simulink model "verify_Storage_Type_11_mdl_electric"  (R2018b)
settings: Solver=VariableStepAuto  StartTime=0  StopTime=9000  MaxStep=60  RelTol=1e-3  EnableMultiTasking=on
undefined symbols (not defined in the file or in its folder): path_carnot
libraries: carnot x10, simulink x5
settings Model: DEBUGGLOBALLEVEL=DEBUGLEVEL  DEBUGMAXTOTALWARNINGS=0  DEBUGMAXCONSECUTIVEWARNINGS=0  DEBUGWRITETOFILE=0  DEBUGFILENAME='error.txt'  Creator=drhf  LastModifiedBy=P41573
settings DataIOCC: SaveFormat=Array
settings OptimizationCC: ExpressionDepthLimit=2147483647  LifeSpan=inf
settings DebuggingCC: UnderspecifiedInitializationDetection=Classic  MergeDetectMultiDrivingBlocksExec=none  SolverPrmCheckMsg=warning  FcnCallInpInsideContextMsg=warning  StateNameClashWarn=warning  SFUnexpectedBacktrackingDiag=warning  SFNoUnconditionalDefaultTransitionDiag=warning  SFExecutionAtInitializationDiag=none
settings HardwareCC: ProdBitPerPointer=32  ProdBitPerSizeT=32  ProdBitPerPtrDiffT=32  ProdLargestAtomicFloat=None  ProdIntDivRoundTo=Undefined  ProdEndianess=Unspecified  ProdWordSize=32  ProdHWDeviceType=32-bit Generic
settings ModelReferenceCC: PropagateSignalLabelsOutOfModel=off
settings SFSimCC: SimUseLocalCustomCode=off
settings RTWCC: RTWUseLocalCustomCode=off
settings CodeAppCC: StateflowObjectComments=on
settings GRTTargetCC: TargetLangStandard=C89/C90 (ANSI)  GeneratePreprocessorConditionals=Disable all  CombineOutputUpdateFcns=off  GRTInterface=on
settings ConfigComp: CovMetricSettings=dw  CovHtmlReporting=on  CovSaveCumulativeToWorkspaceVar=on  CovSaveSingleToWorkspaceVar=on  CovExternalEMLEnable=off

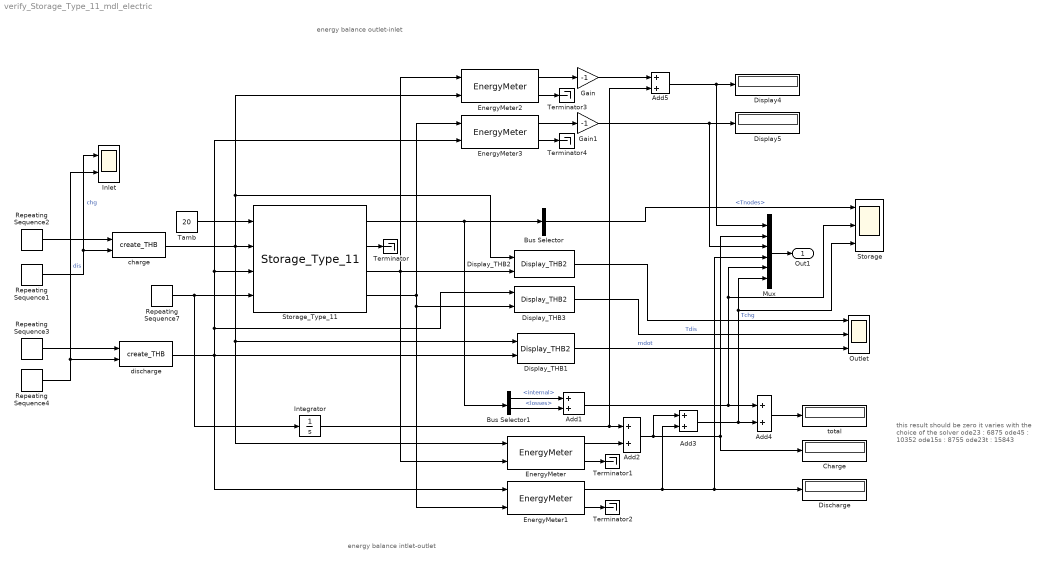
== system verify_Storage_Type_11_mdl_electric ==
  note: this result should be zero
      | it varies with the choice of the solver
      | ode23 : 6875
      | ode45 : 10352
      | ode15s : 8755
      | ode23t : 15843
  note: energy balance outlet-inlet
  note: energy balance intlet-outlet
  Add{1..5} (5 alike) : Sum  Inputs=2
  Bus Selector : BusSelector  OutputSignals=Tnodes
  Bus Selector1 : BusSelector  OutputSignals=energy.internal,energy.losses
  Charge : Display
  Discharge : Display
  Display4 : Display
  Display5 : Display
  Display_THB1 : carnot/Outputs/Display_THB2  t=off  m=on  p=off  id=off  mix=off  d=off
      settings: SourceProductName=Carnot
  Display_THB2 : carnot/Outputs/Display_THB2  t=on  m=off  p=off  id=off  mix=off  d=off
      settings: SourceProductName=Carnot
  Display_THB3 : carnot/Outputs/Display_THB2  t=on  m=off  p=off  id=off  mix=off  d=off
      settings: SourceProductName=Carnot
  EnergyMeter{,1..3} (4 alike) : carnot/Control/EnergyMeter
      settings: SourceProductName=Carnot
  Gain : Gain  Gain=-1
  Gain1 : Gain  Gain=-1
  Inlet : Scope  NumInputPorts=2
  Integrator : Integrator
  Mux : Mux  Inputs=6
  Outlet : Scope  NumInputPorts=3
  Repeating Sequence1 : simulink/Sources/Repeating Sequence  rep_seq_t=[0 1000 1200 1400 9000]  rep_seq_y=[50 50 20 50 50]
  Repeating Sequence2 : simulink/Sources/Repeating Sequence  rep_seq_t=[0 3600 3700 6400 6500 9000]  rep_seq_y=[0.4 0.4 0.1 0.1 0 0]
  Repeating Sequence3 : simulink/Sources/Repeating Sequence  rep_seq_t=[0 3500 3600 9000]  rep_seq_y=[0.1 0.1 0.4 0.4]
  Repeating Sequence4 : simulink/Sources/Repeating Sequence  rep_seq_t=[0 3700 3800 3900 9000]  rep_seq_y=[10 10 40 10 10]
  Repeating Sequence7 : simulink/Sources/Repeating Sequence  rep_seq_t=[ 0 5400 5401 7200 7201]  rep_seq_y="[ 0   0     3e3  3e3     0 ]"
  Storage : Scope  NumInputPorts=3
  Storage_Type_11 : carnot/Storage/Thermal/Storage_Type_11  t0=10  hgt=1.7684  stgtype=11  tini=[10 10 10 10 10 10 10 10 10 10]  mpts=[1 2 3 4 5 6 7 8 9 10]  PathName=fullfile(path_carnot('libsl'), 'Storage', 'Thermal', 'Storage_Type_11', 'parameter_set')  FileName='<user defined>'  userPath=off  userParam=on  uwall=1  ubot=1  utop=1  axcond=1  volume=0.5  dia=0.6  standing=standing cylinder  nodes=10  mpoints=10  Tsensor=0.5  vTpiece=0.004  pipe1inlet=1  pipe1outlet=0  pipe1dia=0.03  pipe2inlet=0.1  pipe2outlet=1  pipe2dia=0.03  heater1start=0.6  heater1end=0.65
      settings: SourceProductName=Carnot
  Tamb : Constant  Value=20
  Terminator{,1..4} (5 alike) : Terminator
  charge : carnot/Source/Simple/create_THB  p=1e5  fluid=Water  mix=0  mix2=0  mix3=0  dia=0  hgt=0  mID=No Pressure Drop
      settings: SourceProductName=Carnot
  discharge : carnot/Source/Simple/create_THB  p=1e5  fluid=Water  mix=0  mix2=0  mix3=0  dia=0  hgt=0  mID=No Pressure Drop
      settings: SourceProductName=Carnot
  total : Display
  Out1 : Outport
  wires:
  Repeating Sequence3/1 -> discharge/1
  Repeating Sequence4/1 -> Inlet/2, discharge/2  "dis"
  EnergyMeter2/2 -> Terminator3/1
  Display_THB1/1 -> Outlet/3  "mdot"
  EnergyMeter3/2 -> Terminator4/1
  Display_THB3/1 -> Outlet/2  "Tdis"
  Add2/1 -> Add3/1, Mux/2, Charge/1
  discharge/1 -> EnergyMeter1/1, Display_THB3/1, EnergyMeter3/2, Storage_Type_11/3, Display_THB1/2
  EnergyMeter1/1 -> Mux/4, Discharge/1, Add3/2
  EnergyMeter/2 -> Terminator1/1
  Display_THB2/1 -> Outlet/1  "Tchg"
  EnergyMeter3/1 -> Gain1/1
  EnergyMeter1/2 -> Terminator2/1
  Repeating Sequence2/1 -> charge/1
  Tamb/1 -> Storage_Type_11/1
  Add1/1 -> Mux/5, Storage/2, Add4/1
  Bus Selector/1 -> Storage/1  "<Tnodes>"
  charge/1 -> Storage_Type_11/2, Display_THB1/1, EnergyMeter/1, Display_THB2/1, EnergyMeter2/2
  Repeating Sequence1/1 -> Inlet/1, charge/2  "chg"
  Storage_Type_11/1 -> Bus Selector/1, Bus Selector1/1
  Storage_Type_11/4 -> EnergyMeter3/1, EnergyMeter1/2, Display_THB3/2
  Storage_Type_11/2 -> Terminator/1
  Storage_Type_11/3 -> EnergyMeter2/1, Display_THB2/2, EnergyMeter/2
  Mux/1 -> Out1/1
  Bus Selector1/2 -> Add1/2  "<losses>"
  Bus Selector1/1 -> Add1/1  "<internal>"
  Add4/1 -> total/1
  Add3/1 -> Storage/3, Mux/6, Add4/2
  Add5/1 -> Mux/1, Display4/1
  Gain1/1 -> Mux/3, Display5/1
  Repeating Sequence7/1 -> Integrator/1, Storage_Type_11/4
  EnergyMeter/1 -> Add2/2
  Integrator/1 -> Add5/2, Add2/1
  EnergyMeter2/1 -> Gain/1
  Gain/1 -> Add5/1
